simulink model "KarnoppNoDet"  (R2018b)
settings: Solver=VariableStepAuto  StartTime=0.0  StopTime=10.0  RelTol=1e-3
libraries: simulink x1
settings Model: Creator=Kjetk  LastModifiedBy=Kjetk

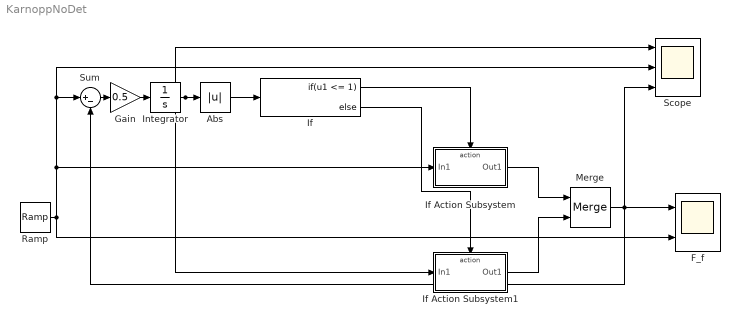
== system KarnoppNoDet ==
  Abs : Abs
  "F_f " : Scope  NumInputPorts=2
  Gain : Gain  Gain=0.5
  If : If  IfExpression=u1 <= 1
  If Action Subsystem : Subsystem  TreatAsAtomicUnit=on
  If Action Subsystem1 : Subsystem  TreatAsAtomicUnit=on
  Integrator : Integrator  InitialCondition=-2
  Merge : Merge
  Ramp : simulink/Sources/Ramp  slope=1  start=0  InitialOutput=0
  Scope : Scope  NumInputPorts=3
  Sum : Sum  Inputs=|+-
  wires:
  If/2 -> If Action Subsystem1/Action
  If/1 -> If Action Subsystem/Action
  Ramp/1 -> If Action Subsystem/1(In1), Sum/1, Scope/2, "F_f "/2
  Integrator/1 -> Scope/1, If Action Subsystem1/1(In1), Abs/1
  Abs/1 -> If/1
  If Action Subsystem/1(Out1) -> Merge/1
  If Action Subsystem1/1(Out1) -> Merge/2
  Merge/1 -> Scope/3, "F_f "/1, Sum/2
  Sum/1 -> Gain/1
  Gain/1 -> Integrator/1

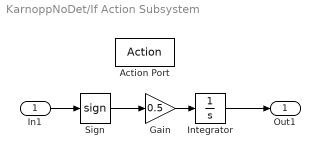
== system KarnoppNoDet/If Action Subsystem ==
  In1 : Inport
  Action Port : ActionPort  ActionType=then
  Gain : Gain  Gain=0.5
  Integrator : Integrator
  Sign : Signum
  Out1 : Outport
  wires:
  In1/1 -> Sign/1
  Sign/1 -> Gain/1
  Gain/1 -> Integrator/1
  Integrator/1 -> Out1/1

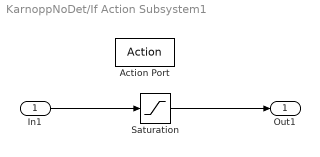
== system KarnoppNoDet/If Action Subsystem1 ==
  In1 : Inport
  Action Port : ActionPort  ActionType=else
  Saturation : Saturate  UpperLimit=1.5  LowerLimit=-1.5
  Out1 : Outport
  wires:
  In1/1 -> Saturation/1
  Saturation/1 -> Out1/1
